simulink model "IndustrialMicrogrid"  (R2023a)
settings: Solver=FixedStepDiscrete  StartTime=0.0  StopTime=10  FixedStep=Ts  RelTol=1e-3
PostLoadFcn:
  | IndustrialMicrogridInputData
  | GfmGridFormingConverterInputParameters
model workspace (MAT data in the model file):
  caseNum = 2
undefined symbols (not defined in the file): base, BESS, DiscIntNeverNeededParam, grid, Grid, gridInverter, machine, microgrid, PV, PVInverter, PVTransformer, scrFactorRg, scrFactorXg, transformer, Ts
libraries: ee_lib x112, eeGeneralControl x104, nesl_utility_internal x64, simulink x56, nesl_utility x37, fl_lib x29, slpidlib x13, eeTransforms x11, eeTotalHarmonicDistorsion x8, eeRmsMeasurement x4, eeSinusoidalMeasurement x4, simulink_extras x2
(part 14 of 14)

== matlab function IndustrialMicrogrid/MG1 Primary Substation/BESS and Controller/BESS/Grid-Forming Converter Control/Measurement/Frequency Measurement/Frequency Measurement/If Action Subsystem/Frequency estimation/MATLAB Function ==
  data: y1 input; y2 input; x1 input; x output; x2 input
function x = fcn(y1,y2,x1,x2)
% Line equation between two points is y-y1=((y2-y1)/(x2-x1))*(x-x1). Here
% to to find the zero crossing instant substitute y = 0 and find x
slope = (y2-y1)/(x2-x1);
x = x1-y1/slope;
